simulink model "QPSK_sim"  (Simulink 7.7)
settings: Solver=VariableStepDiscrete  StartTime=0.0  StopTime=simulationTime  RelTol=1e-3
values from neighbouring files (symbols this model uses):
  lengthOfSymbol = 32    [qpsk_sim_config.m]
  sampleTime = 1    [qpsk_sim_config.m]
undefined symbols (not defined in the file or in its folder): get
libraries: commdigbbndpm3 x5, commchan3 x5, dspsigops x5, commsink2 x3
settings Model: Creator=Philipp Fetzer  LastModifiedBy=mainster
settings DebuggingCC: StrictBusMsg=Warning

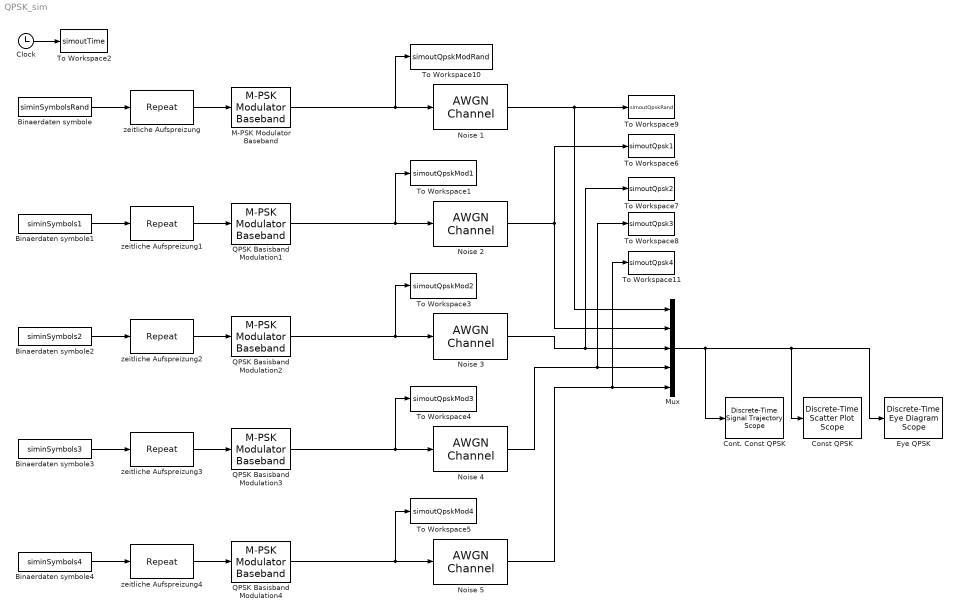
== system QPSK_sim ==
  Binaerdaten symbole : FromWorkspace  VariableName=siminSymbolsRand  SampleTime=sampleTime
  Binaerdaten symbole1 : FromWorkspace  VariableName=siminSymbols1  SampleTime=sampleTime
  Binaerdaten symbole2 : FromWorkspace  VariableName=siminSymbols2  SampleTime=sampleTime
  Binaerdaten symbole3 : FromWorkspace  VariableName=siminSymbols3  SampleTime=sampleTime
  Binaerdaten symbole4 : FromWorkspace  VariableName=siminSymbols4  SampleTime=sampleTime
  Clock : Clock
  Const QPSK : commsink2/Discrete-Time Scatter Plot Scope  Tag=ScatterPlot  SystemSampleTime=-1  sampPerSymb=lengthOfSymbol  offsetEye=0  numTraces=150  numNewFrames=20  LineMarkers=.  LineColors=b  fading=on  render=on  AxisGrid=on  xMin=-1.3  xMax=1.315  yMin=-1.3  yMax=1.315  inphaseLabel=Amplitude Realteil  quadratureLabel=Amplitude Imaginaerteil  openScopeAtSimStart=off  FrameNumber=off  FigPos=get(0,'defaultfigureposition');  figTitle=Konstellationsdiagramm  numLinesMax=8  block_type_=scatter
  Cont. Const QPSK : commsink2/Discrete-Time Signal Trajectory Scope  Tag=SignalTrajectory  SystemSampleTime=-1  sampPerSymb=lengthOfSymbol  offsetEye=0  numTraces=40  numNewFrames=10  LineStyles=-  LineColors=b  fading=on  render=on  AxisGrid=on  xMin=-1.3  xMax=1.315  yMin=-1.3  yMax=1.315  inphaseLabel=Amplitude Realteil  quadratureLabel=Amplitude Imaginaerteil  openScopeAtSimStart=on  FrameNumber=on  FigPos=get(0,'defaultfigureposition');  figTitle=Verlauf Konstellationsdiagramm  numLinesMax=8  block_type_=xy
  Eye QPSK : commsink2/Discrete-Time Eye Diagram Scope  Tag=EyeDiagram  SystemSampleTime=-1  sampPerSymb=lengthOfSymbol  offsetEye=0  symbPerTrace=2  numTraces=40  numNewFrames=10  LineStyles=-  LineColors=b  dupPoints=on  fading=on  render=on  AxisGrid=on  yMin=-1.5  yMax=1.5  inphaseLabel=Amplitude Realteil  quadratureLabel=Amplitude Imaginaerteil  openScopeAtSimStart=off  dispDiagram=In-phase and Quadrature  FrameNumber=off  FigPos=get(0,'defaultfigureposition');  figTitle=Augendiagramm (2 Symbole)  block_type_=eye  numLinesMax=8
  M-PSK Modulator Baseband : commdigbbndpm3/M-PSK Modulator Baseband  M=4  InType=Integer  Enc=Gray  Mapping=[0:7]  Ph=pi/4  outDtype=double  outWordLen=16  outUDDataType=sfix(16)  outFracLenMode=Best precision  outFracLen=15
  Mux : Mux  Inputs=5
  Noise {1..5} (5 alike) : commchan3/AWGN Channel  SystemSampleTime=-1  InputProcessing=Inherited (this choice will be removed - see release notes)  seed=67  noiseMode="Signal to noise ratio  (SNR)"  EbNodB=30  EsNodB=10  SNRdB=SNR  bitsPerSym=1  Ps=1  Tsym=1  variance=1
  QPSK Basisband Modulation{1..4} (4 alike) : commdigbbndpm3/M-PSK Modulator Baseband  M=4  InType=Integer  Enc=Gray  Mapping=[0:2]  Ph=pi/4  outDtype=double  outWordLen=16  outUDDataType=sfix(16)  outFracLenMode=Best precision  outFracLen=15
  To Workspace1 : ToWorkspace  VariableName=simoutQpskMod1  SampleTime=-1  SaveFormat=Structure
  To Workspace10 : ToWorkspace  VariableName=simoutQpskModRand  SampleTime=-1  SaveFormat=Structure
  To Workspace11 : ToWorkspace  VariableName=simoutQpsk4  SampleTime=-1  SaveFormat=Structure
  To Workspace2 : ToWorkspace  VariableName=simoutTime  SampleTime=-1  SaveFormat=Structure
  To Workspace3 : ToWorkspace  VariableName=simoutQpskMod2  SampleTime=-1  SaveFormat=Structure
  To Workspace4 : ToWorkspace  VariableName=simoutQpskMod3  SampleTime=-1  SaveFormat=Structure
  To Workspace5 : ToWorkspace  VariableName=simoutQpskMod4  SampleTime=-1  SaveFormat=Structure
  To Workspace6 : ToWorkspace  VariableName=simoutQpsk1  SampleTime=-1  SaveFormat=Structure
  To Workspace7 : ToWorkspace  VariableName=simoutQpsk2  SampleTime=-1  SaveFormat=Structure
  To Workspace8 : ToWorkspace  VariableName=simoutQpsk3  SampleTime=-1  SaveFormat=Structure
  To Workspace9 : ToWorkspace  VariableName=simoutQpskRand  SampleTime=-1  SaveFormat=Structure
  zeitliche Aufspreizung{,1..4} (5 alike) : dspsigops/Repeat  N=lengthOfSymbol  InputProcessing=Inherited (this choice will be removed - see release notes)  RateOptions=Allow multirate processing  ic=0  mode=Unused parameter value
  wires:
  Clock/1 -> To Workspace2/1
  M-PSK Modulator Baseband/1 -> Noise 1/1, To Workspace10/1
  Binaerdaten symbole/1 -> zeitliche Aufspreizung/1
  QPSK Basisband Modulation1/1 -> Noise 2/1, To Workspace1/1
  QPSK Basisband Modulation2/1 -> Noise 3/1, To Workspace3/1
  Binaerdaten symbole2/1 -> zeitliche Aufspreizung2/1
  zeitliche Aufspreizung2/1 -> QPSK Basisband Modulation2/1
  QPSK Basisband Modulation3/1 -> Noise 4/1, To Workspace4/1
  Binaerdaten symbole3/1 -> zeitliche Aufspreizung3/1
  zeitliche Aufspreizung3/1 -> QPSK Basisband Modulation3/1
  QPSK Basisband Modulation4/1 -> Noise 5/1, To Workspace5/1
  Binaerdaten symbole4/1 -> zeitliche Aufspreizung4/1
  zeitliche Aufspreizung4/1 -> QPSK Basisband Modulation4/1
  Noise 1/1 -> Mux/1, To Workspace9/1
  Noise 2/1 -> Mux/2, To Workspace6/1
  Noise 3/1 -> Mux/3, To Workspace7/1
  Noise 4/1 -> Mux/4, To Workspace8/1
  Noise 5/1 -> Mux/5, To Workspace11/1
  Mux/1 -> Cont. Const QPSK/1, Const QPSK/1, Eye QPSK/1
  Binaerdaten symbole1/1 -> zeitliche Aufspreizung1/1
  zeitliche Aufspreizung1/1 -> QPSK Basisband Modulation1/1
  zeitliche Aufspreizung/1 -> M-PSK Modulator Baseband/1
